simulink model "rtwdemo_lct_inherit_dims"  (Simulink 7.6)
settings: Solver=FixedStepDiscrete  StartTime=0.0  StopTime=10.0  FixedStep=1  RelTol=1e-3
values from neighbouring files (symbols this model uses):
  p1 = Simulink.Parameter    [rtwdemo_capi_data.m]
  p2 = Simulink.Parameter    [rtwdemo_capi_data.m]
  p3 = Simulink.Parameter    [rtwdemo_capi_data.m]
libraries: rtwdemowidgets x2
Description:
  | Inherited Signal Dimensions
settings Model: Creator=The MathWorks Inc.  ExtModeAutoUpdateStatusClock=off
settings MATStruct: SampleTime=1  Offset=0  Priority=[20.0]
settings DataIOCC: SaveOutput=off  SaveTime=off  SignalLoggingName=logsOut
settings OptimizationCC: InlineParams=on  InlineInvariantSignals=on  EfficientFloat2IntCast=on  EfficientMapNaN2IntZero=off
settings DebuggingCC: SolverPrmCheckMsg=none  SignalLabelMismatchMsg=warning  RootOutportRequireBusObject=none  StrictBusMsg=ErrorOnBusTreatedAsVector
settings HardwareCC: ProdIntDivRoundTo=Zero  ProdEndianess=LittleEndian  ProdHWDeviceType=Generic->32-bit Embedded Processor  TargetHWDeviceType=Generic->32-bit Embedded Processor
settings RTWCC: GenerateReport=on  RTWVerbose=off  ProcessScript=grt_make_rtw_hook  LaunchReport=on
settings GRTTargetCC: TargetFcnLib=ansi_tfl_tmw.mat

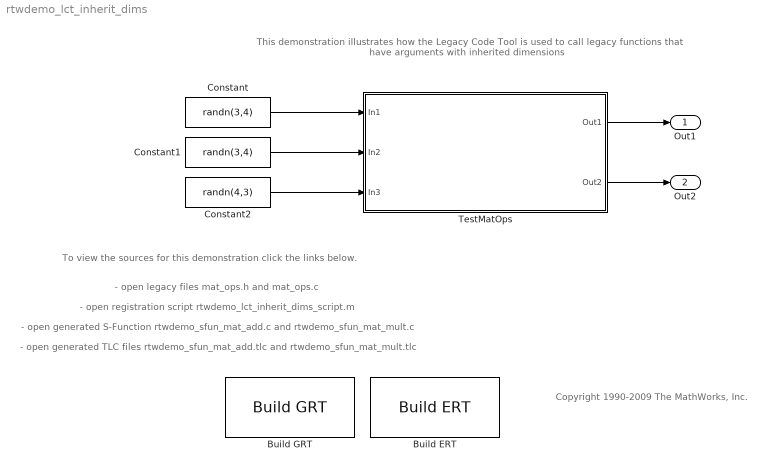
== system rtwdemo_lct_inherit_dims ==
  note: Copyright 1990-2009 The MathWorks, Inc.
  note: This demonstration illustrates how the Legacy Code Tool is used to
      | call legacy functions that have arguments with inherited dimensions
  note: - open legacy files mat_ops.h and mat_ops.c
  note: To view the sources for this demonstration
      | click the links below.
  note: - open registration script rtwdemo_lct_inherit_dims_script.m
  note: - open generated S-Function rtwdemo_sfun_mat_add.c and rtwdemo_sfun_mat_mult.c
  note: - open generated TLC files rtwdemo_sfun_mat_add.tlc and rtwdemo_sfun_mat_mult.tlc
  Build ERT : rtwdemowidgets/Build ERT  SystemSampleTime=-1  attrib_overrides={}
  Build GRT : rtwdemowidgets/Build GRT  SystemSampleTime=-1  attrib_overrides={}
  Constant : Constant  Value=randn(3,4)  OutDataTypeStr=double
  Constant1 : Constant  Value=randn(3,4)  OutDataTypeStr=double
  Constant2 : Constant  Value=randn(4,3)  OutDataTypeStr=double
  TestMatOps : Subsystem
  Out1 : Outport
  Out2 : Outport  Port=2
  wires:
  TestMatOps/1(Out1) -> Out1/1
  Constant/1 -> TestMatOps/1(In1)
  Constant1/1 -> TestMatOps/2(In2)
  Constant2/1 -> TestMatOps/3(In3)
  TestMatOps/2(Out2) -> Out2/1

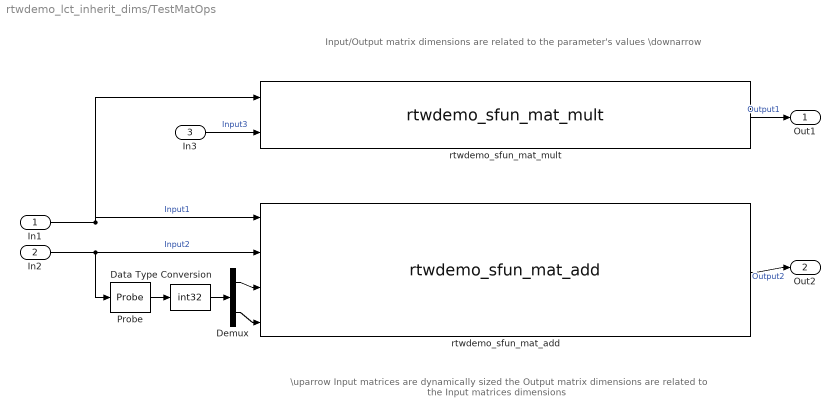
== system rtwdemo_lct_inherit_dims/TestMatOps ==
  note: Input/Output matrix dimensions are related to the parameter's values
      | \downarrow
  note: \uparrow
      | Input matrices are dynamically sized
      | the Output matrix dimensions are related to the Input matrices dimensions
  In1 : Inport
  In2 : Inport  Port=2
  In3 : Inport  Port=3
  Data Type Conversion : DataTypeConversion  OutDataTypeStr=int32
  Demux : Demux  Outputs=2
  Probe : Probe  ProbeWidth=off  ProbeSampleTime=off  ProbeComplexSignal=off  ProbeSignalDimensions=on
  rtwdemo_sfun_mat_add : S-Function  FunctionName=rtwdemo_sfun_mat_add  EnableBusSupport=off  mask(Legacy Function){SFunctionSpec=void mat_add(double u1[][], double u2[][], int32 u3, int32 u4, double y1[size(u1,1)][size(u1,2)]), ShowSpec=on}
      mask prompts: ShowSpec "Display function specification"
      mask help:
      | This block allows you to call the legacy functions specified by the following Legacy Code Tool definition:
      | def.SFunctionName = 'rtwdemo_sfun_mat_add';
      | def.OutputFcnSpec = 'void mat_add(double u1[][], double u2[][], int32 u3, int32 u4, double y1[size(u1,1)][size(u1,2)])';
      | def.HeaderFiles = {'mat_ops.h'};
      | def.SourceFiles = {'mat_ops.c'};
      | def.IncPaths = {'sldemo_lct_src'};
      | def.SrcPaths = {'sldemo_lct_src'};
      mask Help: <p>This block was generated automatically by the Legacy Code Tool. For detailed help on this tool, call<a href="matlab:legacy_code('help')"> legacy_code('help')</a>.</p>
      mask CallbackString:
      | |if strcmp(get_param(gcbh, 'ShowSpec'), 'on')
      |   set_param(gcbh, 'MaskDisplay', sprintf('fprintf(''%s'');', get_param(gcbh, 'SFunctionSpec')));
      | else
      |   set_param(gcbh, 'MaskDisplay', sprintf('fprintf(''%s'');', get_param(gcbh, 'FunctionName')));
      | end
      mask Display: fprintf('void mat_add(double u1[][], double u2[][], int32 u3, int32 u4, double y1[size(u1,1)][size(u1,2)])');
  rtwdemo_sfun_mat_mult : S-Function  FunctionName=rtwdemo_sfun_mat_mult  Parameters=SParameter1, SParameter2, SParameter3  EnableBusSupport=off  mask(Legacy Function){SFunctionSpec=void mat_mult(double u1[p1][p2], double u2[p2][p3], int32 p1, int32 p2, int32 p3, double y1[p1][p3]), SParameter1=int32(3), SParameter2=int32(4), SParameter3=int32(3), ShowSpec=on}
      mask prompts: SParameter1 "P1:"; SParameter2 "P2:"; SParameter3 "P3:"; ShowSpec "Display function specification"
      mask help:
      | This block allows you to call the legacy functions specified by the following Legacy Code Tool definition:
      | def.SFunctionName = 'rtwdemo_sfun_mat_mult';
      | def.OutputFcnSpec = 'void mat_mult(double u1[p1][p2], double u2[p2][p3], int32 p1, int32 p2, int32 p3, double y1[p1][p3])';
      | def.HeaderFiles = {'mat_ops.h'};
      | def.SourceFiles = {'mat_ops.c'};
      | def.IncPaths = {'sldemo_lct_src'};
      | def.SrcPaths = {'sldemo_lct_src'};
      mask Help: <p>This block was generated automatically by the Legacy Code Tool. For detailed help on this tool, call<a href="matlab:legacy_code('help')"> legacy_code('help')</a>.</p>
      mask CallbackString:
      | ||||if strcmp(get_param(gcbh, 'ShowSpec'), 'on')
      |   set_param(gcbh, 'MaskDisplay', sprintf('fprintf(''%s'');', get_param(gcbh, 'SFunctionSpec')));
      | else
      |   set_param(gcbh, 'MaskDisplay', sprintf('fprintf(''%s'');', get_param(gcbh, 'FunctionName')));
      | end
      mask Display: fprintf('void mat_mult(double u1[p1][p2], double u2[p2][p3], int32 p1, int32 p2, int32 p3, double y1[p1][p3])');
  Out1 : Outport
  Out2 : Outport  Port=2
  wires:
  In2/1 -> Probe/1, rtwdemo_sfun_mat_add/2  "Input2"
  rtwdemo_sfun_mat_add/1 -> Out2/1  "Output2"
  In1/1 -> rtwdemo_sfun_mat_add/1, rtwdemo_sfun_mat_mult/1  "Input1"
  Data Type Conversion/1 -> Demux/1
  Probe/1 -> Data Type Conversion/1
  Demux/2 -> rtwdemo_sfun_mat_add/4
  Demux/1 -> rtwdemo_sfun_mat_add/3
  In3/1 -> rtwdemo_sfun_mat_mult/2  "Input3"
  rtwdemo_sfun_mat_mult/1 -> Out1/1  "Output1"
